simulink model "Tanques_NL"  (Simulink 8.3)
settings: Solver=ode45  StartTime=0.0  StopTime=1000.0  RelTol=1e-3
libraries: fuzblock x1
settings Model: Creator=fabiomudearaujo  LastModifiedBy=nildo  NumberOfSteps=100
settings DataIOCC: SignalLoggingSaveFormat=Dataset  InspectSignalLogs=on
settings DebuggingCC: UnderspecifiedInitializationDetection=Simplified  StateNameClashWarn=none
settings GRTTargetCC: CombineOutputUpdateFcns=on  GRTInterface=off

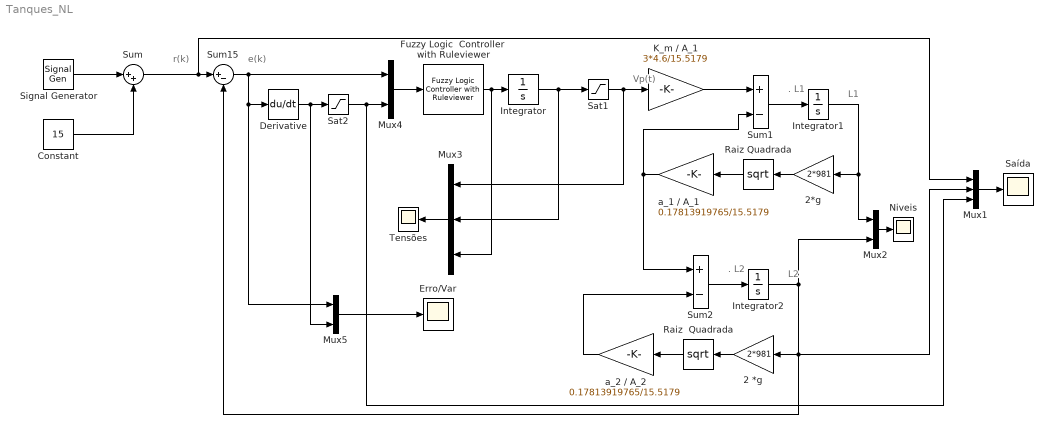
== system Tanques_NL ==
  note: r(k)
  note: .
      | L1
  note: e(k)
  note: Vp(t)
  note: L1
  note: .
      | L2
  note: L2
  2 *g : Gain  Gain=2*981
  2*g : Gain  Gain=2*981
  Constant : Constant  Value=15
  Derivative : Derivative
  Erro/Var : Scope
      settings: TimeRange=500  YMin=0  YMax=30  SaveName=Level1  MaxDataPoints=500000
  Fuzzy Logic  Controller  with Ruleviewer : fuzblock/Fuzzy Logic  Controller  with Ruleviewer  fismatrix=Fuzzy2  Ts=2
  Integrator : Integrator  LimitOutput=on  UpperSaturationLimit=4  LowerSaturationLimit=-4
  Integrator1 : Integrator
  Integrator2 : Integrator
  K_m / A_1 : Gain  Gain=3*4.6/15.5179
  Mux1 : Mux  Inputs=3
  Mux2 : Mux  Inputs=2
  Mux3 : Mux  Inputs=3
  Mux4 : Mux  Inputs=2
  Mux5 : Mux  Inputs=2
  Niveis : Scope
      settings: TimeRange=2000  YMin=-12.5  YMax=27.5  SaveName=Niveis  MaxDataPoints=500000
  Raiz Quadrada : Math  Operator=sqrt  SaturateOnIntegerOverflow=on
  Raiz  Quadrada : Math  Operator=sqrt  SaturateOnIntegerOverflow=on
  Sat1 : Saturate  UpperLimit=4  LowerLimit=-4
  Sat2 : Saturate  UpperLimit=1  LowerLimit=-1
  Saída : Scope
      settings: TimeRange=1000  YMin=-2.5  YMax=22.5  SaveName=Level  MaxDataPoints=500000
  Signal Generator : SignalGenerator  WaveForm=square  Amplitude=5  Frequency=1/(1*240)
  Sum : Sum  Inputs=|++
  Sum1 : Sum  Inputs=+-  SaturateOnIntegerOverflow=on  InputSameDT=on  OutDataTypeStr=Inherit: Same as first input
  Sum15 : Sum  Inputs=|+-  SaturateOnIntegerOverflow=on  InputSameDT=on  OutDataTypeStr=Inherit: Same as first input
  Sum2 : Sum  Inputs=+-  SaturateOnIntegerOverflow=on  InputSameDT=on  OutDataTypeStr=Inherit: Same as first input
  Tensões : Scope
      settings: TimeRange=1000  YMin=-40  YMax=60  SaveName=Vp  MaxDataPoints=500000
  a_1 / A_1 : Gain  Gain=0.17813919765/15.5179
  a_2 / A_2 : Gain  Gain=0.17813919765/15.5179
  wires:
  Sum/1 -> Mux1/1, Sum15/1
  Mux1/1 -> Saída/1
  Mux2/1 -> Niveis/1
  Sat1/1 -> K_m / A_1/1, Mux3/1
  K_m / A_1/1 -> Sum1/1
  Sum1/1 -> Integrator1/1
  Integrator1/1 -> 2*g/1, Mux2/1
  2*g/1 -> Raiz Quadrada/1
  Raiz Quadrada/1 -> a_1 / A_1/1
  a_1 / A_1/1 -> Sum1/2, Sum2/1
  Sum2/1 -> Integrator2/1
  Integrator2/1 -> Mux2/2, 2 *g/1, Sum15/2, Mux1/2
  2 *g/1 -> Raiz  Quadrada/1
  Raiz  Quadrada/1 -> a_2 / A_2/1
  a_2 / A_2/1 -> Sum2/2
  Sum15/1 -> Mux4/1, Mux5/1, Derivative/1
  Mux3/1 -> Tensões/1
  Derivative/1 -> Mux5/2, Sat2/1
  Integrator/1 -> Sat1/1, Mux3/2
  Sat2/1 -> Mux1/3, Mux4/2
  Mux5/1 -> Erro/Var/1
  Constant/1 -> Sum/2
  Signal Generator/1 -> Sum/1
  Mux4/1 -> Fuzzy Logic  Controller  with Ruleviewer/1
  Fuzzy Logic  Controller  with Ruleviewer/1 -> Mux3/3, Integrator/1
